simulink model "Lift"  (R2017a)
settings: Solver=VariableStepAuto  StartTime=0.0  StopTime=10.0  RelTol=1e-3
settings Model: Creator=tlum1  LastModifiedBy=tlum1

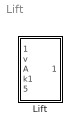
== system Lift ==
  Lift : Subsystem

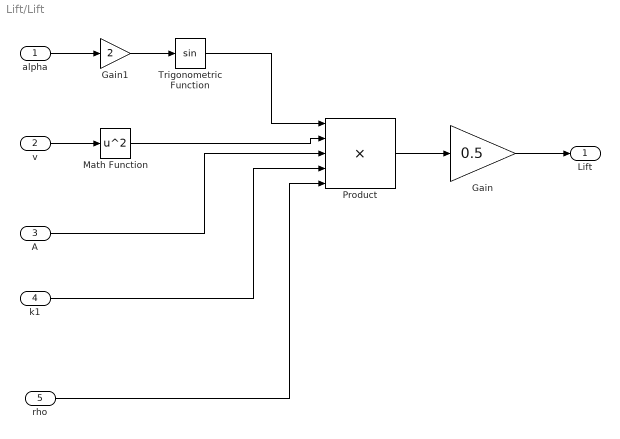
== system Lift/Lift ==
  alpha : Inport
  v : Inport  Port=2
  A : Inport  Port=3
  k1 : Inport  Port=4
  rho : Inport  Port=5
  Gain : Gain  Gain=0.5
  Gain1 : Gain  Gain=2
  Math Function : Math  Operator=square  SaturateOnIntegerOverflow=on
  Product : Product  Inputs=5
  Trigonometric Function : Trigonometry
  Lift : Outport
  wires:
  Gain/1 -> Lift/1
  alpha/1 -> Gain1/1
  Gain1/1 -> Trigonometric Function/1
  Product/1 -> Gain/1
  Math Function/1 -> Product/2
  v/1 -> Math Function/1
  A/1 -> Product/3
  k1/1 -> Product/4
  rho/1 -> Product/5
  Trigonometric Function/1 -> Product/1
